simulink model "RBNN_sys_association_2"  (R2019a)
settings: Solver=FixedStepAuto  StartTime=0.0  StopTime=inf  FixedStep=0.00001  RelTol=1e-3
libraries: dspxfrm3 x1
settings Model: NumberOfSteps=64  Creator=vardhah  LastModifiedBy=vardhah
settings DataIOCC: ReturnWorkspaceOutputs=off
settings DebuggingCC: UnderSpecifiedDimensionMsg=warning  ArithmeticOperatorsInVariantConditions=warning

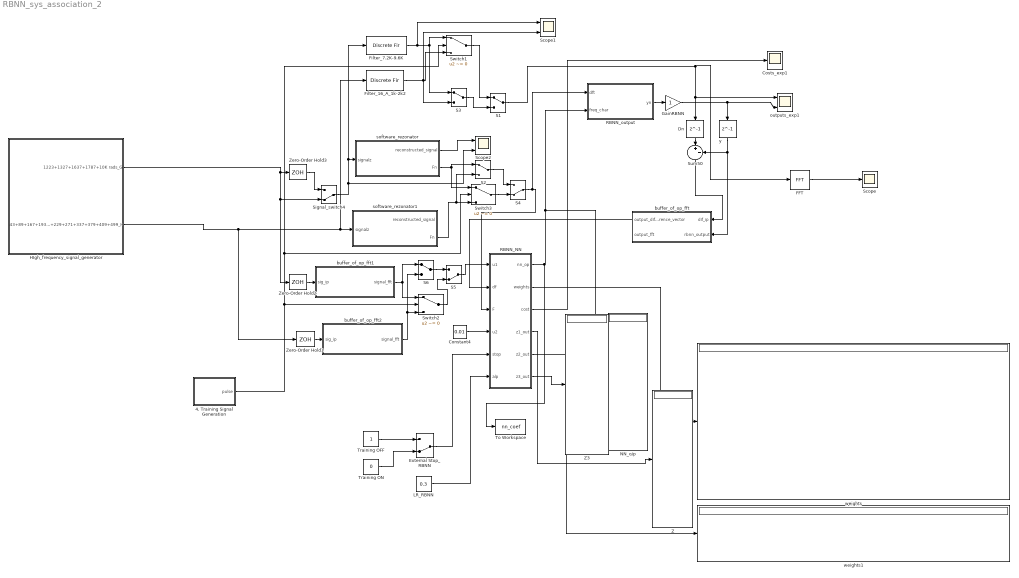
== system RBNN_sys_association_2 ==
  4. Training Signal Generation : MATLAB Function  TreatAsAtomicUnit=on
  Constant4 : Constant  Value=0.01
  Costs_exp1 : Scope
  Dn : Delay  DelayLength=1  InitialCondition=0
  External Stop_RBNN : ManualSwitch  CurrentSetting=0
  FFT : dspxfrm3/FFT  FFTImplementation=Auto  CompMethod=Table lookup  TableOpt=NEW  TableOptActive=Speed  BitRevOrder=off  Normalize=off  InheritFFTLength=off  FFTLength=16  WrapInput=on  roundingMode=Floor  overflowMode=off  firstCoeffDataTypeStr=Inherit: Same word length as input  firstCoeffLastDataTypeStr=Inherit: Same word length as input  outputMin=[]  outputMax=[]
  Filter_16_A_1k-2k2 : DiscreteFir  Tag=BlockMethodSubSystem  Coefficients=[-0.198889914644374777 0.0882189428518377339 0.0736891495871065116 0.0638368801789635787 0.0566372642221577294 0.0523172683654103132 0.0494565343907736044 0.048157521822162791 0.048157521822162791 0.0494565343907736044 0.0523172683654103132 0.0566372642221577294 0.0638368801789635787 0.0736891495871065116 0.0882189428518377339 -0.198889914644374777]  InputProcessing=Columns as channels (frame based)
  "Filter_7.2K-9.6K " : DiscreteFir  Tag=BlockMethodSubSystem  Coefficients=[-0.0120785049852322399 -0.0942455273574688279 0.0101245004695954266 0.125460404555770566 0.034165372769331126 -0.1614987160724079 -0.0984930555982914957 0.150982315564688691 0.150982315564688691 -0.0984930555982914957 -0.1614987160724079 0.034165372769331126 0.125460404555770566 0.0101245004695954266 -0.0942455273574688279 -0.0120785049852322399]  InputProcessing=Columns as channels (frame based)
  GainRBNN : Gain
  HIgh_frequency_signal_generator : Subsystem
  LR_RBNN : Constant  Value=0.3
  NN_o/p : Display
  RBNN_NN : MATLAB Function  TreatAsAtomicUnit=on
  RBNN_output : MATLAB Function  TreatAsAtomicUnit=on
  S{1..3,6} (4 alike) : ManualSwitch
  S4 : ManualSwitch  CurrentSetting=0
  S5 : ManualSwitch  CurrentSetting=0
  Scope : Scope
  Scope1 : Scope  NumInputPorts=2
  Scope2 : Scope  NumInputPorts=2
  Signal_switch4 : ManualSwitch  CurrentSetting=0
  Sum50 : Sum  Inputs=|+-
  Switch1 : Switch  Criteria=u2 ~= 0
  Switch2 : Switch  Criteria=u2 ~= 0
  Switch3 : Switch  Criteria=u2 ~= 0
  To Workspace : ToWorkspace  VariableName=nn_coef  SaveFormat=Timeseries  SampleTime=-1
  Training OFF : Constant
  Training ON : Constant  Value=0
  Z : Display
  Z3 : Display
  Zero-Order Hold1 : ZeroOrderHold  SampleTime=0.00001
  Zero-Order Hold2 : ZeroOrderHold  SampleTime=0.00001
  Zero-Order Hold3 : ZeroOrderHold  SampleTime=0.00001
  buffer_of_op_fft : MATLAB Function  TreatAsAtomicUnit=on
  buffer_of_op_fft1 : MATLAB Function  TreatAsAtomicUnit=on  SystemSampleTime=0.00001
  buffer_of_op_fft2 : MATLAB Function  TreatAsAtomicUnit=on  SystemSampleTime=0.00001
  outputs_exp1 : Scope  NumInputPorts=2
  software_rezonator : MATLAB Function  TreatAsAtomicUnit=on  SystemSampleTime=0.00001
  software_rezonator1 : MATLAB Function  TreatAsAtomicUnit=on  SystemSampleTime=0.00001
  weights : Display
  weights1 : Display
  y : Delay  DelayLength=1  InitialCondition=0
  wires:
  software_rezonator/1(reconstructed_signal) -> Scope2/1
  RBNN_output/1(yn) -> GainRBNN/1
  Dn/1 -> Sum50/1
  y/1 -> buffer_of_op_fft/2(rbnn_output), Sum50/2
  RBNN_NN/1(nn_op) -> To Workspace/1, RBNN_output/2(freq_char), NN_o/p/1
  External Stop_RBNN/1 -> RBNN_NN/5(stop)
  Training OFF/1 -> External Stop_RBNN/1
  Training ON/1 -> External Stop_RBNN/2
  RBNN_NN/3(cost) -> Costs_exp1/1
  RBNN_NN/2(weights) -> weights/1
  RBNN_NN/4(z1_out) -> Z/1
  Sum50/1 -> buffer_of_op_fft/1(dif_ip)
  buffer_of_op_fft/1(output_difference_vector) -> RBNN_NN/2(df)
  S1/1 -> FFT/1, Dn/1, outputs_exp1/1
  LR_RBNN/1 -> RBNN_NN/6(alp)
  GainRBNN/1 -> y/1, outputs_exp1/2
  Signal_switch4/1 -> Scope2/2, "Filter_7.2K-9.6K "/1, software_rezonator/1(signalz)
  Zero-Order Hold3/1 -> Signal_switch4/1
  FFT/1 -> Scope/1
  Switch1/1 -> S1/1
  "Filter_7.2K-9.6K "/1 -> Scope1/1, Switch1/1, S3/1
  Filter_16_A_1k-2k2/1 -> Scope1/2, S3/2, Switch1/3
  4. Training Signal Generation/1(pulse) -> Switch2/2, Switch3/2, Switch1/2
  Constant4/1 -> RBNN_NN/4(u2)
  S3/1 -> S1/2
  HIgh_frequency_signal_generator/2(43+89+167+193+229+271+337+379+409+499_H) -> Zero-Order Hold1/1, Filter_16_A_1k-2k2/1, software_rezonator1/1(signalz)
  RBNN_NN/6(z3_out) -> Z3/1
  RBNN_NN/5(z2_out) -> weights1/1
  software_rezonator/2(Fn) -> Switch3/1, S2/1
  software_rezonator1/2(Fn) -> S2/2, Switch3/3
  Switch3/1 -> S4/2
  S4/1 -> RBNN_output/1(dft), RBNN_NN/3(F)
  S2/1 -> S4/1
  HIgh_frequency_signal_generator/1(1223+1327+1637+1787+10K rads_G) -> Zero-Order Hold2/1, Signal_switch4/2, Zero-Order Hold3/1
  buffer_of_op_fft2/1(signal_fft) -> Switch2/3, S6/2
  Zero-Order Hold1/1 -> buffer_of_op_fft2/1(sig_ip)
  Zero-Order Hold2/1 -> buffer_of_op_fft1/1(sig_ip)
  buffer_of_op_fft1/1(signal_fft) -> Switch2/1, S6/1
  S6/1 -> S5/1
  Switch2/1 -> S5/2
  S5/1 -> RBNN_NN/1(u1)

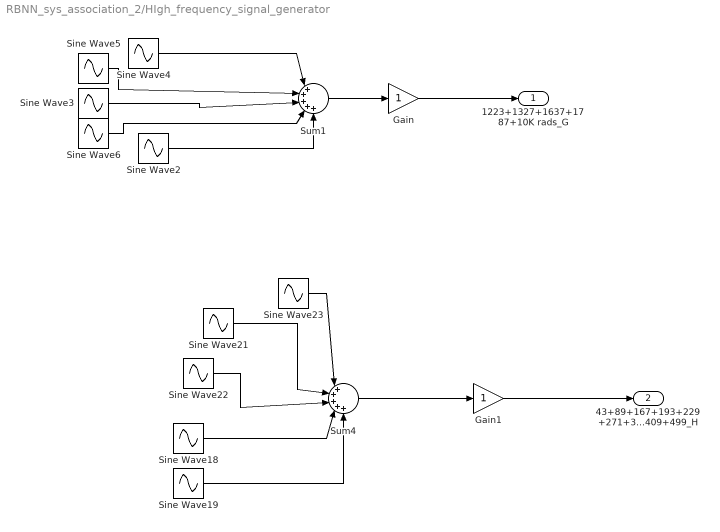
== system RBNN_sys_association_2/HIgh_frequency_signal_generator ==
  Gain : Gain
  Gain1 : Gain
  Sine Wave18 : Sin  Amplitude=0.2  Frequency=409  SampleTime=0
  Sine Wave19 : Sin  Amplitude=0.2  Frequency=499  SampleTime=0
  Sine Wave2 : Sin  Frequency=1000  SampleTime=0
  Sine Wave21 : Sin  Amplitude=0  Frequency=337  SampleTime=0
  Sine Wave22 : Sin  Amplitude=0.2  Frequency=379  SampleTime=0
  Sine Wave23 : Sin  Amplitude=0  Frequency=271  SampleTime=0
  Sine Wave3 : Sin  Frequency=2000  SampleTime=0
  Sine Wave4 : Sin  Frequency=50  SampleTime=0
  Sine Wave5 : Sin  Frequency=100  SampleTime=0
  Sine Wave6 : Sin  Frequency=1787  SampleTime=0
  Sum1 : Sum  Inputs=|+++++
  Sum4 : Sum  Inputs=|+++++
  1223+1327+1637+1787+10K rads_G : Outport
  43+89+167+193+229+271+337+379+409+499_H : Outport  Port=2
  wires:
  Sine Wave23/1 -> Sum4/1
  Sine Wave22/1 -> Sum4/3
  Sine Wave18/1 -> Sum4/4
  Sine Wave19/1 -> Sum4/5
  Sine Wave5/1 -> Sum1/2
  Sine Wave4/1 -> Sum1/1
  Sine Wave21/1 -> Sum4/2
  Sine Wave6/1 -> Sum1/4
  Sine Wave2/1 -> Sum1/5
  Sine Wave3/1 -> Sum1/3
  Sum1/1 -> Gain/1
  Sum4/1 -> Gain1/1
  Gain/1 -> 1223+1327+1637+1787+10K rads_G/1
  Gain1/1 -> 43+89+167+193+229+271+337+379+409+499_H/1

== matlab function RBNN_sys_association_2/software_rezonator1 ==
  data: signalz input; reconstructed_signal output; Fn output size=16
function [reconstructed_signal,Fn]   = rezonator(signalz)

persistent numberofrezonator;
persistent g c bfr_rezo_sm aft_delay dft_out;
persistent out signal_dif;
persistent n;
persistent memory_alloc_flag;


%assign the number of rezonator here. For configuring it for higher order
%rezonator  we need to change (1) 'numberofrezonaotor' variable
if isempty(numberofrezonator)
        numberofrezonator = 16;   %here 16 parallel rezonators
end
N=16;
%Initialisation of memory allocations/variables ====> 
if isempty(memory_alloc_flag)
        memory_alloc_flag = 0; 
end
if isempty(g)
       g=zeros(numberofrezonator,numberofrezonator,'like',0i); 
end
if isempty(c)
       c=zeros(numberofrezonator,numberofrezonator,'like',0i); 
end
if memory_alloc_flag==0
 for i=0:numberofrezonator-1
  for j= 0:numberofrezonator-1
   g(i+1,j+1)=1/numberofrezonator*(exp(-1i*2*pi*i*j/numberofrezonator));
   c(i+1,j+1)=(exp(1i*2*pi*i*j/numberofrezonator));
  end 
 end
 memory_alloc_flag=1;
end


%Initialisation of variables  =====> 
if isempty(n)
        n = 0;   
end 
if isempty(out)
  out=0+0i;
end
if isempty(signal_dif)
  signal_dif=0+0i;
end
if isempty(bfr_rezo_sm)
  bfr_rezo_sm=repmat(0+0i,numberofrezonator,1);
end
if isempty(aft_delay)
  aft_delay=repmat(0+0i,numberofrezonator,1);
end
if isempty(dft_out)
  dft_out=repmat(0+0i,numberofrezonator,1);
end

%creating cycle of rotation for selection of correct column of g & c.
cycle=mod(n,numberofrezonator);

%resonator core -----------------------------> 
dft_out=c(:,cycle+1).*aft_delay;
out= sum(dft_out,1);
signal_dif=signalz-out;
bfr_rezo_sm=g(:,cycle+1).*signal_dif;

%counting the counter
n=n+1;

% output assignment ------------------>
reconstructed_signal=out;
dft=aft_delay; 
%N=size(dft,1);
a=1:1:N/2-1;
b=N/2+1:1:N-1;
dft_trans=transpose(dft);
Fn=transpose([real(dft_trans(1)) 2*(real(dft_trans(2:N/2)).*cos(2*pi*a*n/N)-imag(dft_trans(2:N/2)).*sin(2*pi*a*n/N)) -1^n*real(dft_trans(N/2+1)) -2*(imag(dft_trans(N/2+2:N)).*cos(2*pi*b*n/N)+real(dft_trans(N/2+2:N)).*sin(2*pi*b*n/N))]);
%--------output assignment over----------<

%final updation of buffer ------>>>>>>>>>>>>
aft_delay= aft_delay+bfr_rezo_sm; 
end

== matlab function RBNN_sys_association_2/RBNN_NN ==
  settings: sampleTime=0.01
  data: u1 input; df input; F input; u2 input; nn_op output; weights output; cost output; z1_out output; stop input; alp input; z2_out output; z3_out output
function [nn_op,weights,cost,z1_out,z2_out,z3_out]  = NN(u1,df,F,u2,stop,alp)

persistent w1 w2 w3;
persistent vy;
persistent g1 g2 g3;
persistent itr;
persistent J;
persistent del_w1 del_w2 del_w3;
persistent mult1 mult2 mult3;
persistent memory_alloc_flag;
persistent n;
persistent z1 z2 z3 an3;
%%
%%%%%%----------------------------------------------------------------------------%%%%%
%Hyper-parameter & other tunable part of code

M=16;   %declare batch size of training (It will also be equal to number of input in our case as we are using DFT)
E=1;    % size of external associative input

%layer declaration
layer_1=32;
layer_2=64;
layer_3=16;       % Output layer must match with number of rezonators declared in rezonator function

%learning rate. Currently reading from input pin 
alpha = alp;

%others
input_layer =M+E;       %layer_0
output_layer=layer_3;

% weight Intialisation 
if isempty(w1)
       w1=randn(input_layer,layer_1)*0.1;
end
if isempty(w2)
       w2=randn(layer_1,layer_2)*0.1;
end
if isempty(w3)
       w3=randn(layer_2,layer_3)*0.1;
end

%%%%%---------------------------------------------------------------------------------%%%%%

%%

%synchronising clock
if isempty(n)
        n = 0; end
n=n+1;

%%
%Allocation of variables that will be used during runtime( one time execution code) 
if isempty(z1)
       z1= zeros(layer_1,1);
end
if isempty(z2)
       z2= zeros(layer_2,1);
end
if isempty(z3)
       z3= zeros(layer_3,1);
end
if isempty(an3)
       an3= zeros(layer_3,1);
end

if isempty(memory_alloc_flag)
        memory_alloc_flag = 0; 
end
if isempty(mult1)
       mult1=zeros(layer_1,layer_1*input_layer); 
end
if isempty(mult2)
       mult2=zeros(layer_2,layer_1*layer_2); 
end
if isempty(mult3)
       mult3=zeros(layer_3,layer_2*layer_3); 
end
if isempty(vy)
       vy=zeros(input_layer,M); 
end

if memory_alloc_flag==0
 %write memory allocation for looped code here.It runs once and store it in memory.  
 mult1=[];
 mult2=[];
 mult3=[];
  for iteration =1:layer_1
   mult1=[mult1;[zeros(1,(iteration-1)*input_layer) ones(1,input_layer) zeros(1,(layer_1-iteration)*input_layer)]];
  end
  for iterate=1:layer_2
   mult2=[mult2;[zeros(1,(iterate-1)*layer_1) ones(1,layer_1) zeros(1,(layer_2-iterate)*layer_1)]];
  end
  for iterate=1:layer_3
   mult3=[mult3;[zeros(1,(iterate-1)*layer_2) ones(1,layer_2) zeros(1,(layer_3-iterate)*layer_2)]];
  end
 %{
 for k= 1:input_layer
    for j = 1:M 
        if k<=(M/2)+1 && k>=1
            vy(k,j)=(1/M)*cos(pi*(M-j)*(k-1)/(M/2));
        elseif k<=M && k>=(M/2)+1
            vy(k,j)=-(1/M)*sin(pi*(M-j)*(k-1)/(M/2));
        elseif k>M
            vy(k,j)=0;     
        end
    end
 end
  %}
 memory_alloc_flag=1; 
end

%%
%============All other Initiaisation =========================>

%Initialisation of delta of weight storage
if isempty(del_w1)
    del_w1=zeros(1,input_layer*layer_1);
end
if isempty(del_w2)
    del_w2=zeros(1,layer_2*layer_1);
end
if isempty(del_w3)
    del_w3=zeros(1,layer_2*layer_3);
end

%Intialising iteration number & cost value. 
if isempty(itr)
    itr=0;
end
if isempty(J)
    J=0;
end


%gradient initialisation(in matrix form)
if isempty(g1)
    g1= zeros(M,input_layer*layer_1);   
end
if isempty(g2)
    g2= zeros(M,layer_1*layer_2);   
end
if isempty(g3)
    g3= zeros(M,layer_3*layer_2);   
end

%%
%Input vector creation code block
x_in = [real(u1(1:(size(u1,2)/2)+1)) imag(u1(1:(size(u1,2)/2)-1))];
v=transpose([x_in transpose(u2)]);

%v=transpose([u1 u2]);
%%
%RBNN core vectorised algorithm implementation 

%--------------->forward propogation ------------>
if sum(1*(max(z3-5,0)>0),'all')==0
 z1=w1'*v ;
%a1=(1./(1+exp(-z1)));
%an1=(a1-0.5);
a1=max(z1,0)+0.1*min(0,z1);
z2=w2'*a1 ;
%z2=w2'*an1 ;
%a2=(1./(1+exp(-z2)));
%an2=(a2-0.5);
a2=max(z2,0)+0.1*min(0,z2);
%z3=w3'*an2 ;
z3=w3'*a2 ;
a3=(1./(1+exp(-z3)));
an3=(a3-0.5)*10;

%-------------> Backward Propogation -------->

%calculation of Nv:
da3_z3=a3.*(1-a3)*10;
dn_a2=w3'.*repmat(da3_z3,1,layer_2);
%da2_z2=a2.*(1-a2);
da2_z2=(1*(a2>=0) + 0.1*((a2>=0)==0));
dn_z2= dn_a2.* repmat(transpose(da2_z2),output_layer,1);
dn_a1=dn_z2*w2';
%da1_z1=a1.*(1-a1); 
da1_z1=(1*(a1>=0) + 0.1*((a1>=0)==0));
dn_z1=dn_a1.*repmat(transpose(da1_z1),output_layer,1);
dn_v=dn_z1*w1';   %"This is Nv" 

%calculation of aD, A & B 
aD=transpose(F)*dn_v*vy;
A=[aD;eye(M-1) zeros(M-1,1)];
B=[transpose(F) ; zeros(M-1,size(F,1))]; 

%calculation of Nw(diff of N(v,w) wrt each weights)
dIn_3= da3_z3*transpose(a2);
dn_w3=repmat(dIn_3,1,layer_3).* mult3;

dIn_2= da2_z2*transpose(a1);
da2_w2=repmat(dIn_2,1,layer_2).* mult2;
dn_w2=dn_a2*da2_w2;

dIn_1= da1_z1*transpose(v);
da1_w1= repmat(dIn_1,1,layer_1).*mult1;
dn_w1=dn_a1*da1_w1;

%gradient updation
g3=A*g3+B*dn_w3;
g2=A*g2+B*dn_w2;
g1=A*g1+B*dn_w1;

%Training & updation only once in a batch(batch size=M,n=Overall counter) 
if mod(n,M)==0 && stop==0 && sum(1*(max(z3-5,0)>0),'all')==0
    del_w1 =alpha*df*1*g1/M ;
    del_w2 =alpha*df*1*g2/M ;
    del_w3 =alpha*df*1*g3/M ;
    del_w_reshaped1= reshape(del_w1,[input_layer,layer_1]);
    del_w_reshaped2= reshape(del_w2,[layer_1,layer_2]);
    del_w_reshaped3= reshape(del_w3,[layer_2,layer_3]);
    w1=w1+ del_w_reshaped1;
    w2=w2+ del_w_reshaped2;
    w3=w3+ del_w_reshaped3; 
    itr=itr+1;
  
end
end
%For logging & visulisation purpose
J= sum(df.^2,'all')/(2*M);
cost=J;
weights=w1;
z1_out=z1;
z2_out=z2;
z3_out=z3;





%NN output assignment
nn_op=an3;


end

== matlab function RBNN_sys_association_2/buffer_of_op_fft ==
  data: output_difference_vector output size=[1,16]; output_fft output size=[1,16]; dif_ip input; rbnn_output input
function [output_difference_vector,output_fft] = difBuffer(dif_ip,rbnn_output)                      

 sz=16;                       % size of the dft 
 
 persistent a;
 persistent b;
 if isempty(b)
  b= zeros(1,sz);
 end
 if isempty(a)
  a= zeros(1,sz);
 end
 
 
  a= circshift(a,1);
  a(1)=dif_ip;
  b= circshift(b,1);
  b(1)=rbnn_output;

 output_difference_vector=a; 
 output_fft=1/sz*fft(b); 
end

== matlab function RBNN_sys_association_2/buffer_of_op_fft1 ==
  data: signal_fft output size=[1,16]; sig_ip input
function signal_fft  = difBuffer(sig_ip)                      

 sz=16;                       % size of the dft 
 
 persistent a;

 if isempty(a)
  a= zeros(1,sz);
 end
 
 
 a= circshift(a,1);
 a(1)=sig_ip;
 
 signal_fft=0.01*1/sz*fft(a); 
end

== matlab function RBNN_sys_association_2/buffer_of_op_fft2 ==
  data: signal_fft output size=[1,16]; sig_ip input
function signal_fft  = difBuffer(sig_ip)                      

 sz=16;                       % size of the dft 
 
 persistent a;

 if isempty(a)
  a= zeros(1,sz);
 end
 
 
 a= circshift(a,1);
 a(1)=sig_ip;
 
 signal_fft=1/sz*fft(a); 
end

== matlab function RBNN_sys_association_2/software_rezonator ==
  data: signalz input; reconstructed_signal output; Fn output size=16
function [reconstructed_signal,Fn]   = rezonator(signalz)

persistent numberofrezonator;
persistent g c bfr_rezo_sm aft_delay dft_out;
persistent out signal_dif;
persistent n;
persistent memory_alloc_flag;


%assign the number of rezonator here. For configuring it for higher order
%rezonator  we need to change (1) 'numberofrezonaotor' variable
if isempty(numberofrezonator)
        numberofrezonator = 16;   %here 16 parallel rezonators
end
N=16;
%Initialisation of memory allocations/variables ====> 
if isempty(memory_alloc_flag)
        memory_alloc_flag = 0; 
end
if isempty(g)
       g=zeros(numberofrezonator,numberofrezonator,'like',0i); 
end
if isempty(c)
       c=zeros(numberofrezonator,numberofrezonator,'like',0i); 
end
if memory_alloc_flag==0
 for i=0:numberofrezonator-1
  for j= 0:numberofrezonator-1
   g(i+1,j+1)=1/numberofrezonator*(exp(-1i*2*pi*i*j/numberofrezonator));
   c(i+1,j+1)=(exp(1i*2*pi*i*j/numberofrezonator));
  end 
 end
 memory_alloc_flag=1;
end


%Initialisation of variables  =====> 
if isempty(n)
        n = 0;   
end 
if isempty(out)
  out=0+0i;
end
if isempty(signal_dif)
  signal_dif=0+0i;
end
if isempty(bfr_rezo_sm)
  bfr_rezo_sm=repmat(0+0i,numberofrezonator,1);
end
if isempty(aft_delay)
  aft_delay=repmat(0+0i,numberofrezonator,1);
end
if isempty(dft_out)
  dft_out=repmat(0+0i,numberofrezonator,1);
end

%creating cycle of rotation for selection of correct column of g & c.
cycle=mod(n,numberofrezonator);

%resonator core -----------------------------> 
dft_out=c(:,cycle+1).*aft_delay;
out= sum(dft_out,1);
signal_dif=signalz-out;
bfr_rezo_sm=g(:,cycle+1).*signal_dif;

%counting the counter
n=n+1;

% output assignment ------------------>
reconstructed_signal=out;
dft=aft_delay; 
%N=size(dft,1);
a=1:1:N/2-1;
b=N/2+1:1:N-1;
dft_trans=transpose(dft);
Fn=transpose([real(dft_trans(1)) 2*(real(dft_trans(2:N/2)).*cos(2*pi*a*n/N)-imag(dft_trans(2:N/2)).*sin(2*pi*a*n/N)) -1^n*real(dft_trans(N/2+1)) -2*(imag(dft_trans(N/2+2:N)).*cos(2*pi*b*n/N)+real(dft_trans(N/2+2:N)).*sin(2*pi*b*n/N))]);
%--------output assignment over----------<

%final updation of buffer ------>>>>>>>>>>>>
aft_delay= aft_delay+bfr_rezo_sm; 
end

== matlab function RBNN_sys_association_2/RBNN_output ==
  data: dft input; yn output; freq_char input
function yn = fcn(dft,freq_char)
yn=transpose(freq_char)*dft;
end

== matlab function RBNN_sys_association_2/4. Training Signal Generation ==
  data: pulse output
function pulse    = fcn
M=64;

persistent cnt;
persistent n;
if isempty(cnt)
    cnt=0;
end
if isempty(n)
    n=0;
end
n=n+1;
if mod(n,M)==0
     cnt=cnt+1;
 end
 pulse = mod(cnt,2);

end
